simulink model "Modelo_Matematico"  (R2021a)
settings: Solver=ode45  StartTime=0.0  StopTime=10  RelTol=1e-3
values from neighbouring files (symbols this model uses):
  b = 0.005752    [Parametros_Modelo.m]
  f = 60    [Parametros_Modelo.m]
  J = 0.02    [Parametros_Modelo.m]
  Kcj = 1/40    (= 0.025)    [Parametros_Modelo.m]
  Lm = 0.2037    [Parametros_Modelo.m]
  Lr = 0.005974    [Parametros_Modelo.m]
  Ls = 0.005974    [Parametros_Modelo.m]
  p = 2    [Parametros_Modelo.m]
  Rr = 1.083    [Parametros_Modelo.m]
  Rs = 1.115    [Parametros_Modelo.m]
settings Model: Creator=electronica  LastModifiedBy=hubertdelgado
settings DebuggingCC: UnconnectedInputMsg=none  UnconnectedOutputMsg=none  UnconnectedLineMsg=none
settings ModelReferenceCC: EnableRefExpFcnMdlSchedulingChecks=off
settings RTWCC: Description=Generic Real-Time Target  DLArmComputeVersion=20.02.1

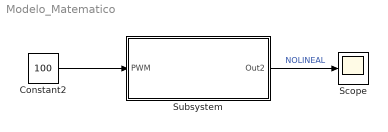
== system Modelo_Matematico ==
  Constant2 : Constant  Value=100
  Scope : Scope
  Subsystem : Subsystem
  wires:
  Constant2/1 -> Subsystem/1(PWM)
  Subsystem/1(Out2) -> Scope/1  "NOLINEAL"

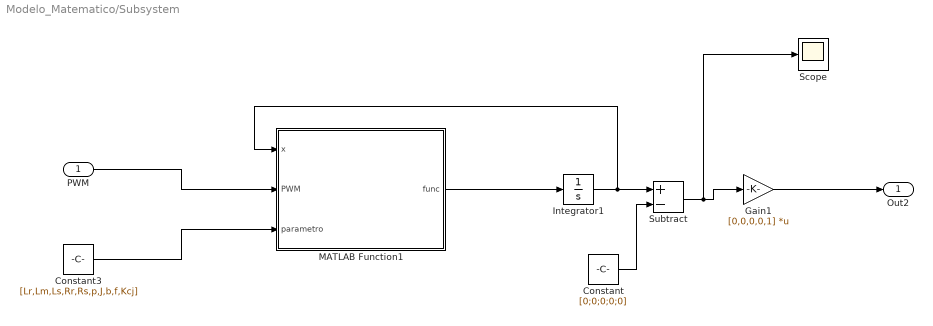
== system Modelo_Matematico/Subsystem ==
  PWM : Inport
  Constant : Constant  Value=[0;0;0;0;0]
  Constant3 : Constant  Value=[Lr,Lm,Ls,Rr,Rs,p,J,b,f,Kcj]
  Gain1 : Gain  Gain=[0,0,0,0,1]  Multiplication=Matrix(K*u)
  Integrator1 : Integrator  InitialCondition=[0;0;0;0;0]
  MATLAB Function1 : MATLAB Function  TreatAsAtomicUnit=on
  Scope : Scope
  Subtract : Sum  Inputs=+-
  Out2 : Outport
  wires:
  PWM/1 -> MATLAB Function1/2(PWM)
  Integrator1/1 -> Subtract/1, MATLAB Function1/1(x)
  Constant3/1 -> MATLAB Function1/3(parametro)
  MATLAB Function1/1(func) -> Integrator1/1
  Subtract/1 -> Scope/1, Gain1/1
  Constant/1 -> Subtract/2
  Gain1/1 -> Out2/1

== matlab function Modelo_Matematico/Subsystem/MATLAB Function1 ==
  data: x input; func output; PWM input; parametro input
function func = fcn(x,PWM,parametro)
%Parametros
Lr = parametro(1);
Lm = parametro(2);
Ls = parametro(3);
Rr = parametro(4);
Rs = parametro(5);
p = parametro(6);
J = parametro(7);
b = parametro(8);
f = parametro(9);
Kcj = parametro(10);

%Estados
Ids = x(1);
Iqs = x(2);
Idr = x(3);
Iqr = x(4);
wm = x(5);

delta = (Lr+Lm)*(Ls+Lm)-Lm^2;
ws = 2*pi*(f*PWM/100);
R = [Rs 0 0 0;
      0 Rs 0 0;
      0 0 Rr 0;
      0 0 0 Rr];

omega = [0, -ws, 0, 0;
    ws, 0, 0, 0;
    0, 0, 0, -(ws-(p*wm));
    0, 0, (ws-(p*wm)), 0];

L = [Ls+Lm, 0, Lm, 0;
    0, Ls+Lm 0, Lm;
    Lm, 0, Lr+Lm, 0;
    0, Lm, 0, Lr+Lm];

% inv_L = (1/delta)*[Lr+Lm, 0, -Lm, 0;
%                   0, Lr+Lm, 0, -Lm;
%                   -Lm, 0, Ls+Lm, 0;
%                   0, -Lm, 0, Ls+Lm];

Vqs = 4.889*(f*PWM/100)+16.15;
V = [Vqs;
       0;
       0;
       0];

I = [Ids;
    Iqs;
    Idr;
    Iqr];

dI = -(inv(L)*R + inv(L)*omega*L)*I + inv(L)*V;
Te = 1.5*p*Lm*(Iqs*Idr - Ids*Iqr);
dwm = (p/J)*(Te - (b)*wm);
func = [dI; dwm];
